simulink model "ELEC448_lab2_dif_kin"  (R2022a)
settings: Solver=ode4  StartTime=0.0  StopTime=inf  FixedStep=0.002  RelTol=1e-3  EnableMultiTasking=on
undefined symbols (not defined in the file or in its folder): HIL, qc_get_step_size
libraries: quarc_library x8
settings Model: ExtModeTrigDuration=10000  Creator=17stf1  LastModifiedBy=19jelg
settings SolverCC: AlgebraicLoopSolver=TrustRegion  PositivePriorityOrder=on
settings DataIOCC: ReturnWorkspaceOutputs=off
settings DebuggingCC: UnconnectedInputMsg=warning  UnconnectedOutputMsg=warning  UnconnectedLineMsg=warning  SFMachineParentedDataDiag=warning  ArithmeticOperatorsInVariantConditions=warning
settings SFSimCC: SimUseLocalCustomCode=off  CustomCodeUndefinedFunction=UseInterfaceOnly
settings RTWCC: Description=QUARC Win64 Target Using Toolchain  SystemTargetFile=quarc_win64.tlc  TemplateMakefile=quarc_default_tmf  RTWUseLocalCustomCode=off  Toolchain=QUARC win64 | nmake (64-bit Windows)  BuildConfiguration=Faster Runs
settings CodeAppCC: StateflowObjectComments=on
settings STFCustomTargetCC: TargetLangStandard=C99 (ISO)  ConcurrentExecutionCompliant=on  UseToolchainInfoCompliant=on  SystemTargetFile=quarc_win64.tlc
settings GRTTargetCC: ParMdlRefBuildCompliant=off  CompOptLevelCompliant=off  CombineOutputUpdateFcns=off  MatFileLogging=off  CPPClassGenCompliant=off  GRTInterface=on  ExtMode=on  ExtModeMexFile=quarc_comm
settings ConfigComp: CovMetricSettings=dswe

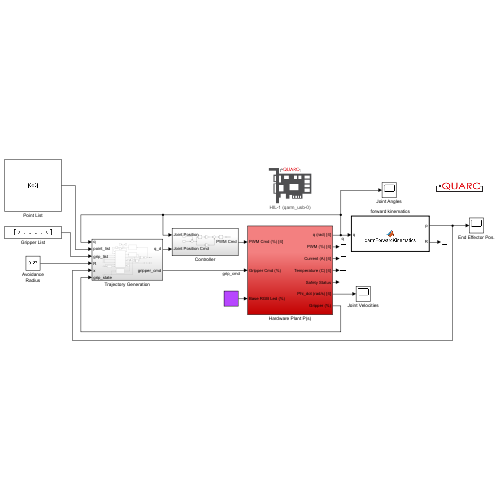
[thumbnail: Simulink's stored preview of the top-level diagram]
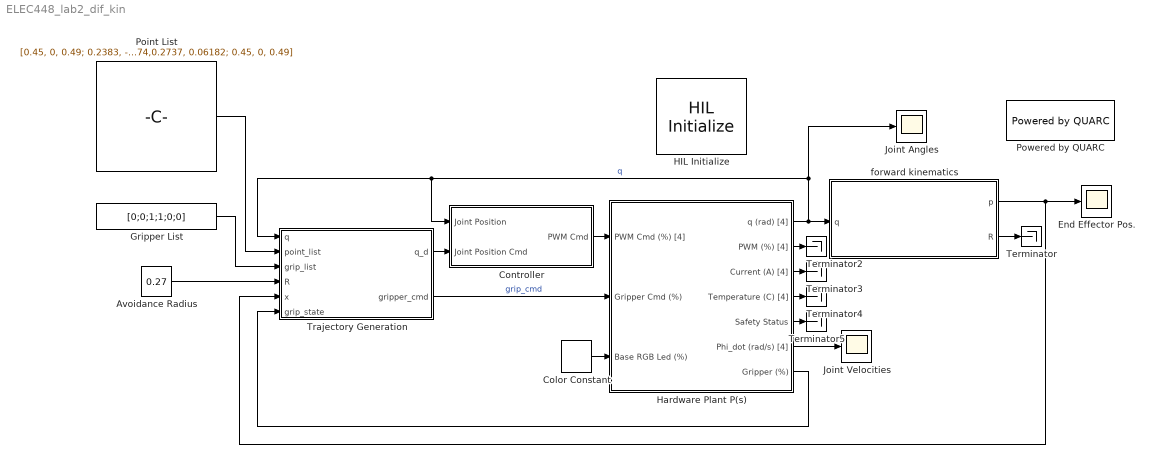
== system ELEC448_lab2_dif_kin ==
  Avoidance Radius : Constant  Value=0.27
  Color Constant : quarc_library/Sources/Signals/Color Constant  color=[0.71765 0.27451 1]
      settings: SourceProductName=QUARC Targets
  Controller : Subsystem
  End Effector Pos. : Scope
  Gripper List : Constant  Value=[0;0;1;1;0;0]
  HIL Initialize : quarc_library/Data Acquisition/Generic/Configuration/HIL Initialize  object_name=HIL-1  board_type=qarm_usb  board_number=0  board_options=j0_mode=1;j1_mode=1;j2_mode=1;j3_mode=1;gripper_mode=0;j0_profile_config=0;j0_profile_velocity=1.5708;j0_profile_acceleration=1.0472;j1_profile_config=0;j1_profile_velocity=1.5708;j1_profile_acceleration=1.0472;j2_profile_config=0;j2_profile_velocity=1.5708;j2_profile_acceleration=1.0472;j3_profile_config=0;j3_profile_velocity=1.5708;j3_profile_acceleration=1.0472;  exclusive=off  active=on  hardware_clocks=[0]  clock_modes=[]  initial_clock_frequencies=[]  set_clock_params_at_start=off  set_clock_params_at_switch_in=off  set_clock_frequencies_at_start=off  set_clock_frequencies_at_switch_in=off  analog_input_channels=[0:9]  analog_input_configurations=[]  analog_input_maximums=5  analog_input_minimums=0  set_analog_input_params_at_start=off  set_analog_input_params_at_switch_in=off  analog_output_channels=[]  analog_output_maximums=[]  analog_output_minimums=[]  initial_analog_outputs=[]  final_analog_outputs=[]  watchdog_analog_outputs=[]  set_analog_output_params_at_start=off  set_analog_output_params_at_switch_in=off  set_analog_outputs_at_start=off  set_analog_outputs_at_switch_in=off  set_analog_outputs_at_terminate=off  set_analog_outputs_at_switch_out=off  set_analog_outputs_on_watchdog=off  digital_input_channels=[]  digital_output_channels=[]  digital_output_configuration=[]  initial_digital_outputs=[0]  final_digital_outputs=[0]  watchdog_digital_outputs=[0]  set_digital_output_params_at_start=off  set_digital_output_params_at_switch_in=off  set_digital_outputs_at_start=on  set_digital_outputs_at_switch_in=off  set_digital_outputs_at_terminate=on  set_digital_outputs_at_switch_out=off  set_digital_outputs_on_watchdog=on  encoder_channels=[]  quadrature=[4]  encoder_filter_frequency=[]  initial_encoder_counts=[0]  set_encoder_params_at_start=off  set_encoder_params_at_switch_in=off  set_encoder_counts_at_start=on  set_encoder_counts_at_switch_in=off  pwm_channels=[]  pwm_modes=[0]  pwm_frequency=50  pwm_configuration=[0]  pwm_alignment=[0]  pwm_polarity=[1]  pwm_leading_deadband=[]  pwm_trailing_deadband=[]  initial_pwm_outputs=[0]  final_pwm_outputs=[0]  watchdog_pwm_outputs=[0]  set_pwm_params_at_start=on  set_pwm_params_at_switch_in=off  set_pwm_outputs_at_start=on  set_pwm_outputs_at_switch_in=off  set_pwm_outputs_at_terminate=on  set_pwm_outputs_at_switch_out=off  set_pwm_outputs_on_watchdog=on  other_output_channels=[1000:1004 11000:11008]  initial_other_outputs=[0]  final_other_outputs=[0]  watchdog_other_outputs=[0]  set_other_outputs_at_start=on  set_other_outputs_at_switch_in=off  set_other_outputs_at_terminate=on  set_other_outputs_at_switch_out=off  set_other_outputs_on_watchdog=on
  Hardware Plant P(s) : Subsystem
  Joint Angles : Scope
  Joint Velocities : Scope
  Point List : Constant  Value=[0.45, 0, 0.49; 0.2383, -0.2831, 0.1474; 0.2379, -0.2736, 0.06678; 0.2593, 0.2566, 0.1446; 0.2574,0.2737, 0.06182; 0.45, 0, 0.49]  VectorParams1D=off
  Powered by QUARC : quarc_library/Logos/Powered by QUARC
  Terminator{,2..5} (5 alike) : Terminator
  Trajectory Generation : Subsystem
  forward kinematics : MATLAB Function  TreatAsAtomicUnit=on
  wires:
  Color Constant/1 -> Hardware Plant P(s)/3(Base RGB Led (%))
  Controller/1(PWM Cmd) -> Hardware Plant P(s)/1(PWM Cmd (%) [4])
  forward kinematics/2(R) -> Terminator/1
  Hardware Plant P(s)/1(q (rad) [4]) -> Joint Angles/1, Controller/1(Joint Position), Trajectory Generation/1(q), forward kinematics/1(q)  "q"
  Trajectory Generation/2(gripper_cmd) -> Hardware Plant P(s)/2(Gripper Cmd (%))  "grip_cmd"
  Hardware Plant P(s)/2(PWM (%) [4]) -> Terminator2/1
  Hardware Plant P(s)/3(Current (A) [4]) -> Terminator3/1
  Hardware Plant P(s)/4(Temperature (C) [4]) -> Terminator4/1
  Hardware Plant P(s)/5(Safety Status) -> Terminator5/1
  Avoidance Radius/1 -> Trajectory Generation/4(R)
  Point List/1 -> Trajectory Generation/2(point_list)
  Gripper List/1 -> Trajectory Generation/3(grip_list)
  Trajectory Generation/1(q_d) -> Controller/2(Joint Position Cmd)
  forward kinematics/1(p) -> Trajectory Generation/5(x), End Effector Pos./1
  Hardware Plant P(s)/7(Gripper (%)) -> Trajectory Generation/6(grip_state)
  Hardware Plant P(s)/6(Phi_dot (rad/s) [4]) -> Joint Velocities/1

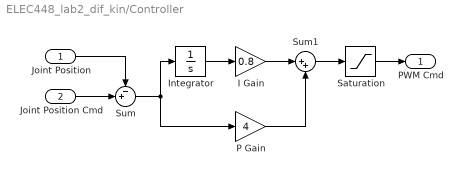
== system ELEC448_lab2_dif_kin/Controller ==
  Joint Position : Inport
  Joint Position Cmd : Inport  Port=2
  I Gain : Gain  Gain=0.8
  Integrator : Integrator  LimitOutput=on  UpperSaturationLimit=0.25  LowerSaturationLimit=-0.25
  P Gain : Gain  Gain=4
  Saturation : Saturate
  Sum : Sum  Inputs=-+|
  Sum1 : Sum  Inputs=|++
  PWM Cmd : Outport
  wires:
  Saturation/1 -> PWM Cmd/1
  Joint Position/1 -> Sum/1
  Joint Position Cmd/1 -> Sum/2
  Integrator/1 -> I Gain/1
  Sum/1 -> P Gain/1, Integrator/1
  Sum1/1 -> Saturation/1
  P Gain/1 -> Sum1/2
  I Gain/1 -> Sum1/1

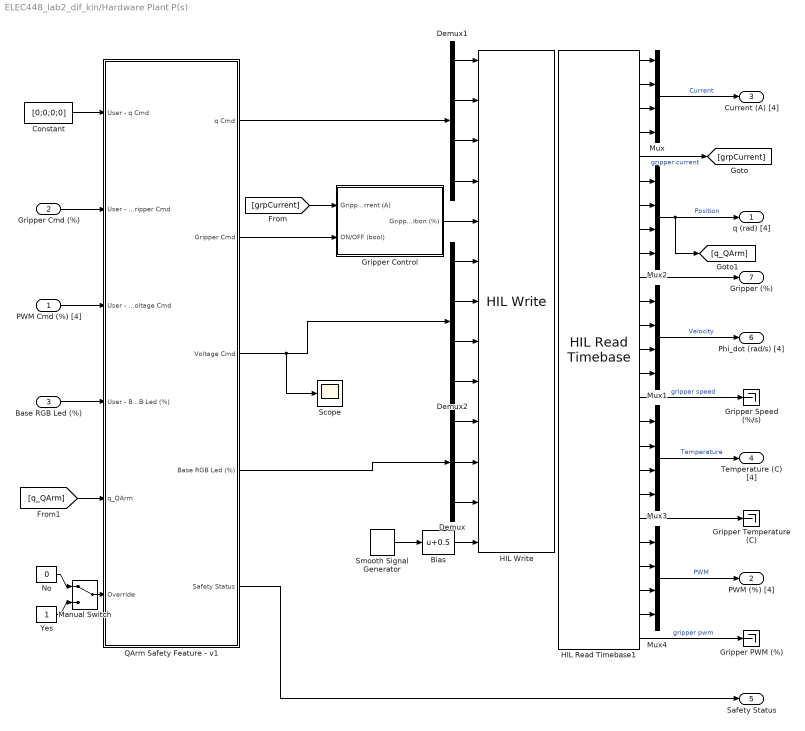
== system ELEC448_lab2_dif_kin/Hardware Plant P(s) ==
  PWM Cmd (%) [4] : Inport
  Gripper Cmd (%) : Inport  Port=2
  Base RGB Led (%) : Inport  Port=3
  Bias : Bias  Bias=0.5  SaturateOnIntegerOverflow=off
  Constant : Constant  Value=[0;0;0;0]
  Demux : Demux  Outputs=3
  Demux1 : Demux
  Demux2 : Demux
  Gripper Control : Subsystem
  Gripper PWM (%) : Terminator
  Gripper Speed (%/s) : Terminator
  Gripper Temperature (C) : Terminator
  HIL Read Timebase1 : quarc_library/Data Acquisition/Generic/Timebases/HIL Read Timebase  object_name=HIL-1  clock=0  analog_channels=[5:9]  encoder_channels=[]  digital_channels=[]  other_channels=[1000:1004 3000:3004 10000:10004 11000:11004]  active=on  vector_output=off  data_type_mode=Inherit via back propagation  encoder_data_type=double  digital_data_type=boolean  overflow_mode=Error on overflow  samples_in_buffer=max(ceil(1/qc_get_step_size), 1)
  HIL Write : quarc_library/Data Acquisition/Generic/Immediate I//O/HIL Write  object_name=HIL-1  analog_channels=[]  pwm_channels=[]  digital_channels=[]  other_channels=[1000:1004 11000:11003 11005:11008]  sample_time=-1  active=on  vector_input=off
  Manual Switch : ManualSwitch
  Mux{,1..4} (5 alike) : Mux
  No : Constant  Value=0
  QArm Safety Feature - v1 : Subsystem
  Scope : Scope
  Smooth Signal Generator : quarc_library/Sources/Signals/Smooth Signal Generator  signal_type=Sine  source=Internal (dialog parameters)  amplitude=0.5  frequency=0.5  initial_phase=0  sample_time=qc_get_step_size  output_cos=off
      settings: SourceProductName=QUARC Targets
  Yes : Constant
  q (rad) [4] : Outport  VectorParamsAs1DForOutWhenUnconnected=off
  PWM (%) [4] : Outport  Port=2  VectorParamsAs1DForOutWhenUnconnected=off
  Current (A) [4] : Outport  Port=3  VectorParamsAs1DForOutWhenUnconnected=off
  Temperature (C) [4] : Outport  Port=4  VectorParamsAs1DForOutWhenUnconnected=off
  Safety Status : Outport  Port=5  VectorParamsAs1DForOutWhenUnconnected=off
  Phi_dot (rad/s) [4] : Outport  Port=6  VectorParamsAs1DForOutWhenUnconnected=off
  Gripper (%) : Outport  Port=7  VectorParamsAs1DForOutWhenUnconnected=off
  wires:
  QArm Safety Feature - v1/2(Gripper Cmd) -> Gripper Control/2(ON/OFF (bool))
  HIL Read Timebase1/10 -> Gripper (%)/1
  Mux4/1 -> PWM (%) [4]/1  "PWM"
  HIL Read Timebase1/25 -> Gripper PWM (%)/1  "gripper pwm"
  HIL Read Timebase1/24 -> Mux4/4
  HIL Read Timebase1/23 -> Mux4/3
  HIL Read Timebase1/22 -> Mux4/2
  HIL Read Timebase1/21 -> Mux4/1
  Demux2/4 -> HIL Write/9
  Demux2/3 -> HIL Write/8
  Demux2/2 -> HIL Write/7
  Demux2/1 -> HIL Write/6
  PWM Cmd (%) [4]/1 -> QArm Safety Feature - v1/3(User - Voltage Cmd)
  Constant/1 -> QArm Safety Feature - v1/1(User - q Cmd)
  Demux1/4 -> HIL Write/4
  Demux1/3 -> HIL Write/3
  Demux1/2 -> HIL Write/2
  Demux1/1 -> HIL Write/1
  Mux3/1 -> Temperature (C) [4]/1  "Temperature"
  Mux1/1 -> Phi_dot (rad/s) [4]/1  "Velocity"
  Mux/1 -> Current (A) [4]/1  "Current"
  HIL Read Timebase1/20 -> Gripper Temperature (C)/1
  HIL Read Timebase1/1 -> Mux/1
  HIL Read Timebase1/2 -> Mux/2
  HIL Read Timebase1/13 -> Mux1/3
  Demux/2 -> HIL Write/11
  HIL Read Timebase1/19 -> Mux3/4
  Demux/1 -> HIL Write/10
  HIL Read Timebase1/11 -> Mux1/1
  HIL Read Timebase1/16 -> Mux3/1
  HIL Read Timebase1/17 -> Mux3/2
  HIL Read Timebase1/3 -> Mux/3
  Demux/3 -> HIL Write/12
  HIL Read Timebase1/15 -> Gripper Speed (%/s)/1  "gripper speed"
  HIL Read Timebase1/5 -> [grpCurrent]  "gripper current"
  HIL Read Timebase1/7 -> Mux2/2
  HIL Read Timebase1/4 -> Mux/4
  HIL Read Timebase1/12 -> Mux1/2
  HIL Read Timebase1/8 -> Mux2/3
  HIL Read Timebase1/18 -> Mux3/3
  HIL Read Timebase1/6 -> Mux2/1
  HIL Read Timebase1/9 -> Mux2/4
  HIL Read Timebase1/14 -> Mux1/4
  Smooth Signal Generator/1 -> Bias/1
  Bias/1 -> HIL Write/13
  Gripper Control/1(Gripper Position (%)) -> HIL Write/5
  [grpCurrent] -> Gripper Control/1(Gripper Current (A))
  [q_QArm] -> QArm Safety Feature - v1/5(q_QArm)
  Yes/1 -> Manual Switch/2
  Manual Switch/1 -> QArm Safety Feature - v1/6(Override)
  No/1 -> Manual Switch/1
  QArm Safety Feature - v1/5(Safety Status) -> Safety Status/1
  QArm Safety Feature - v1/1(q Cmd) -> Demux1/1
  Mux2/1 -> [q_QArm], q (rad) [4]/1  "Position"
  QArm Safety Feature - v1/4(Base RGB Led (%)) -> Demux/1
  Base RGB Led (%)/1 -> QArm Safety Feature - v1/4(User - Base RGB Led (%))
  Gripper Cmd (%)/1 -> QArm Safety Feature - v1/2(User - Gripper Cmd)
  QArm Safety Feature - v1/3(Voltage Cmd) -> Demux2/1, Scope/1

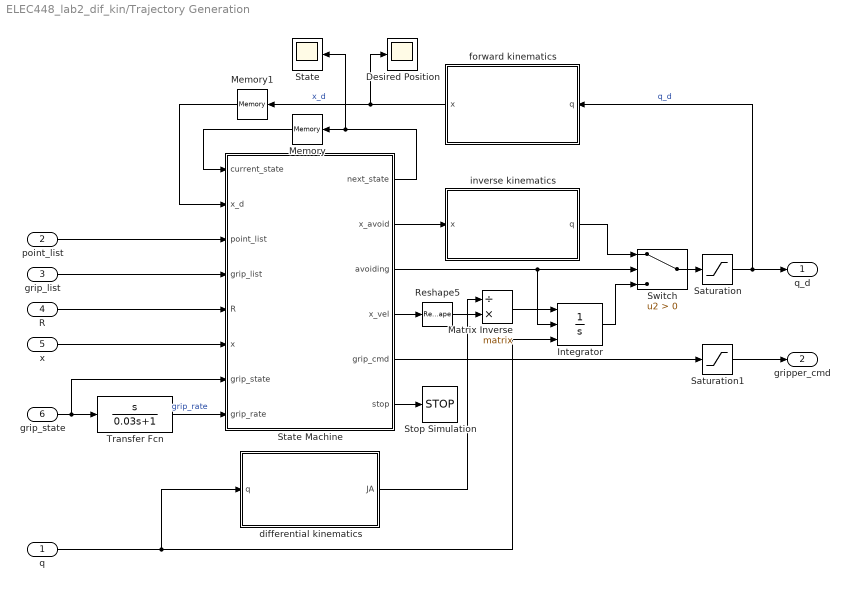
== system ELEC448_lab2_dif_kin/Trajectory Generation ==
  q : Inport
  point_list : Inport  Port=2
  grip_list : Inport  Port=3
  R : Inport  Port=4
  x : Inport  Port=5
  grip_state : Inport  Port=6
  Desired Position : Scope
  Integrator : Integrator  ExternalReset=level  InitialConditionSource=external  UpperSaturationLimit=[170 85 85 180]*pi/180  LowerSaturationLimit=[-170 -85 -95 -180]*pi/180
  Matrix Inverse : Product  Inputs=/*  Multiplication=Matrix(*)
  Memory : Memory  InitialCondition=1
  Memory1 : Memory  InitialCondition=1
  Reshape5 : Reshape  OutputDimensionality=Column vector (2-D)
  Saturation : Saturate  UpperLimit=[170; 85; 75; 167.5]*pi/180  LowerLimit=-[170; 85; 95; 167.5]*pi/180
  Saturation1 : Saturate  UpperLimit=1  LowerLimit=0
  State : Scope
  State Machine : MATLAB Function  TreatAsAtomicUnit=on  SystemSampleTime=0.002
  Stop Simulation : Stop
  Switch : Switch  Criteria=u2 > Threshold  SaturateOnIntegerOverflow=off  InputSameDT=off
  Transfer Fcn : TransferFcn  Numerator=[1 0]  Denominator=[0.03 1]
  differential kinematics : MATLAB Function  TreatAsAtomicUnit=on
  forward kinematics : MATLAB Function  TreatAsAtomicUnit=on
  inverse kinematics : MATLAB Function  TreatAsAtomicUnit=on
  q_d : Outport
  gripper_cmd : Outport  Port=2
  wires:
  forward kinematics/1(x) -> Memory1/1, Desired Position/1  "x_d"
  point_list/1 -> State Machine/3(point_list)
  Memory/1 -> State Machine/1(current_state)
  q/1 -> Integrator/3, differential kinematics/1(q)
  State Machine/4(x_vel) -> Reshape5/1
  R/1 -> State Machine/5(R)
  differential kinematics/1(JA) -> Matrix Inverse/1
  Matrix Inverse/1 -> Integrator/1
  Integrator/1 -> Switch/3
  Saturation/1 -> q_d/1, forward kinematics/1(q)  "q_d"
  State Machine/5(grip_cmd) -> Saturation1/1
  x/1 -> State Machine/6(x)
  Reshape5/1 -> Matrix Inverse/2
  Saturation1/1 -> gripper_cmd/1
  grip_state/1 -> State Machine/7(grip_state), Transfer Fcn/1
  Switch/1 -> Saturation/1
  State Machine/3(avoiding) -> Switch/2, Integrator/2
  State Machine/2(x_avoid) -> inverse kinematics/1(x)
  inverse kinematics/1(q) -> Switch/1
  Memory1/1 -> State Machine/2(x_d)
  State Machine/1(next_state) -> State/1, Memory/1
  grip_list/1 -> State Machine/4(grip_list)
  State Machine/6(stop) -> Stop Simulation/1
  Transfer Fcn/1 -> State Machine/8(grip_rate)  "grip_rate"

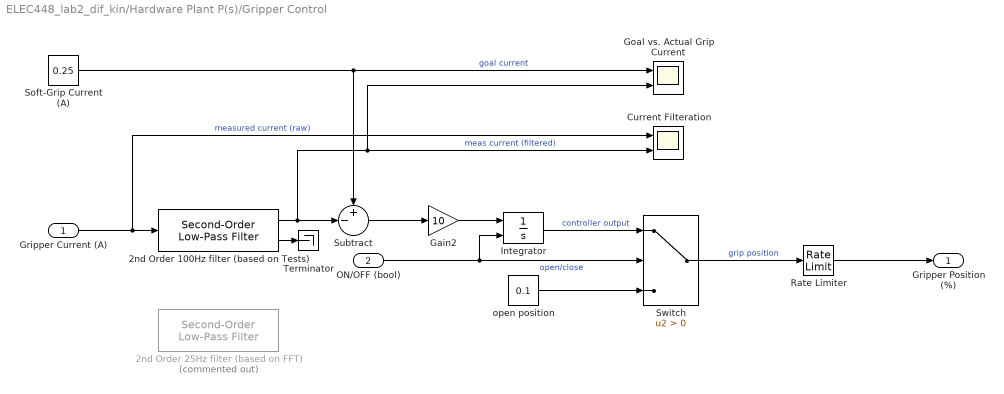
== system ELEC448_lab2_dif_kin/Hardware Plant P(s)/Gripper Control ==
  Gripper Current (A) : Inport
  ON/OFF (bool) : Inport  Port=2
  2nd Order 100Hz filter (based on Tests) : quarc_library/Continuous/Second-Order Low-Pass Filter  params_source=Internal (dialog parameters)  input_width=100*2*pi  input_zeta=1  input_init=0
  2nd Order 25Hz filter (based on FFT) : quarc_library/Continuous/Second-Order Low-Pass Filter  Commented=on  params_source=Internal (dialog parameters)  input_width=25*2*pi  input_zeta=1  input_init=0
  Current Filteration : Scope  NumInputPorts=2
  Gain2 : Gain  Gain=10
  Goal vs. Actual Grip Current : Scope  NumInputPorts=2
  Integrator : Integrator  ExternalReset=either  InitialCondition=0.1  LimitOutput=on  UpperSaturationLimit=0.9  LowerSaturationLimit=0.1
  Rate Limiter : RateLimiter  SampleTimeMode=inherited
  Soft-Grip Current (A) : Constant  Value=0.25
  Subtract : Sum  Inputs=+-|
  Switch : Switch  Criteria=u2 > Threshold  SaturateOnIntegerOverflow=off  InputSameDT=off
  Terminator : Terminator
  open position : Constant  Value=0.1
  Gripper Position (%) : Outport  VectorParamsAs1DForOutWhenUnconnected=off
  wires:
  Gripper Current (A)/1 -> 2nd Order 100Hz filter (based on Tests)/1, Current Filteration/1  "measured current (raw)"
  ON/OFF (bool)/1 -> Switch/2, Integrator/2  "open/close"
  open position/1 -> Switch/3
  Switch/1 -> Rate Limiter/1  "grip position"
  Soft-Grip Current (A)/1 -> Subtract/1, Goal vs. Actual Grip Current/1  "goal current"
  2nd Order 100Hz filter (based on Tests)/1 -> Subtract/2, Current Filteration/2, Goal vs. Actual Grip Current/2  "meas current (filtered)"
  Subtract/1 -> Gain2/1
  Integrator/1 -> Switch/1  "controller output"
  Gain2/1 -> Integrator/1
  2nd Order 100Hz filter (based on Tests)/2 -> Terminator/1
  Rate Limiter/1 -> Gripper Position (%)/1

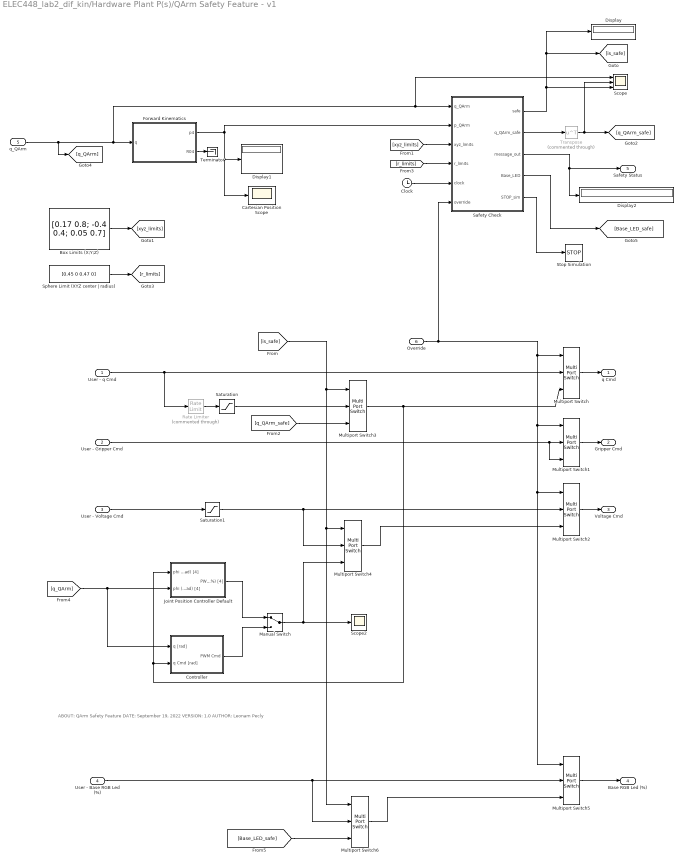
== system ELEC448_lab2_dif_kin/Hardware Plant P(s)/QArm Safety Feature - v1 ==
  note: ABOUT: QArm Safety Feature
      |
      | DATE: September 19, 2022
      |
      | VERSION: 1.0
      |
      | AUTHOR: Leonam Pecly
  User - q Cmd : Inport
  User - Gripper Cmd : Inport  Port=2
  User - Voltage Cmd : Inport  Port=3
  User - Base RGB Led (%) : Inport  Port=4
  q_QArm : Inport  Port=5
  Override : Inport  Port=6
  Box Limits (X;Y;Z) : Constant  Value=[0.17 0.8; -0.4 0.4; 0.05 0.7]
  Cartesian Position Scope : Scope
  Clock : Clock
  Controller : Subsystem
  Display : Display
  Display1 : Display
  Display2 : Display
  Forward Kinematics : MATLAB Function  TreatAsAtomicUnit=on
  Joint Position Controller Default : Subsystem
  Manual Switch : ManualSwitch
  Multiport Switch{,1..6} (7 alike) : MultiPortSwitch  Inputs=2  SaturateOnIntegerOverflow=off  InputSameDT=off
  Rate Limiter : RateLimiter  Commented=through  RisingSlewLimit=pi/2*[1 1 1 2]  FallingSlewLimit=-pi/2*[1 1 1 2]  SampleTimeMode=inherited
  Safety Check : MATLAB Function  TreatAsAtomicUnit=on  SystemSampleTime=qc_get_step_size
  Saturation : Saturate  UpperLimit=pi*[170 85 75 167.5]/180  LowerLimit=pi*[-170 -85 -95 -167.5]/180
  Saturation1 : Saturate  UpperLimit=[1 1 1 1]  LowerLimit=-1*[1 1 1 1]
  Scope : Scope  NumInputPorts=3
  Scope2 : Scope
  Sphere Limit (XYZ center | radius) : Constant  Value=[0.45 0 0.47 0]
  Stop Simulation : Stop
  Terminator : Terminator
  Transpose : Math  Commented=through  Operator=transpose
  q Cmd : Outport
  Gripper Cmd : Outport  Port=2
  Voltage Cmd : Outport  Port=3
  Base RGB Led (%) : Outport  Port=4
  Safety Status : Outport  Port=5
  wires:
  Multiport Switch/1 -> q Cmd/1
  q_QArm/1 -> Scope/1, Safety Check/1(q_QArm), Forward Kinematics/1(q), [q_QArm]
  User - Gripper Cmd/1 -> Multiport Switch1/3, Multiport Switch1/2
  Multiport Switch1/1 -> Gripper Cmd/1
  Multiport Switch2/1 -> Voltage Cmd/1
  User - Voltage Cmd/1 -> Saturation1/1
  Forward Kinematics/1(p4) -> Cartesian Position Scope/1, Display1/1, Safety Check/2(p_QArm)
  [xyz_limits] -> Safety Check/3(xyz_limits)
  Safety Check/1(safe) -> Scope/3, [is_safe], Display/1
  Clock/1 -> Safety Check/5(clock)
  [is_safe] -> Multiport Switch4/1, Multiport Switch6/1, Multiport Switch3/1
  Override/1 -> Safety Check/6(override), Multiport Switch5/1, Multiport Switch2/1, Multiport Switch1/1, Multiport Switch/1
  Box Limits (X;Y;Z)/1 -> [xyz_limits]
  Safety Check/3(message_out) -> Display2/1, Safety Status/1
  [q_QArm] -> Joint Position Controller Default/2(phi (rad) [4]), Controller/1(q [rad])
  User - q Cmd/1 -> Rate Limiter/1, Multiport Switch/2
  Multiport Switch4/1 -> Multiport Switch2/3
  Saturation1/1 -> Multiport Switch2/2, Multiport Switch4/2
  Safety Check/2(q_QArm_safe) -> Transpose/1
  [q_QArm_safe] -> Multiport Switch3/3
  Transpose/1 -> Scope/2, [q_QArm_safe]
  Sphere Limit (XYZ center | radius)/1 -> [r_limits]
  [r_limits] -> Safety Check/4(r_limits)
  Joint Position Controller Default/1(PWM (%) [4]) -> Manual Switch/1
  Controller/1(PWM Cmd) -> Manual Switch/2
  Manual Switch/1 -> Scope2/1, Multiport Switch4/3
  Multiport Switch3/1 -> Multiport Switch/3, Joint Position Controller Default/1(phi cmd (rad) [4]), Controller/2(q Cmd [rad])
  Rate Limiter/1 -> Saturation/1
  Saturation/1 -> Multiport Switch3/2
  Multiport Switch5/1 -> Base RGB Led (%)/1
  User - Base RGB Led (%)/1 -> Multiport Switch5/2, Multiport Switch6/2
  Safety Check/4(Base_LED) -> [Base_LED_safe]
  [Base_LED_safe] -> Multiport Switch6/3
  Multiport Switch6/1 -> Multiport Switch5/3
  Safety Check/5(STOP_sim) -> Stop Simulation/1
  Forward Kinematics/2(R04) -> Terminator/1

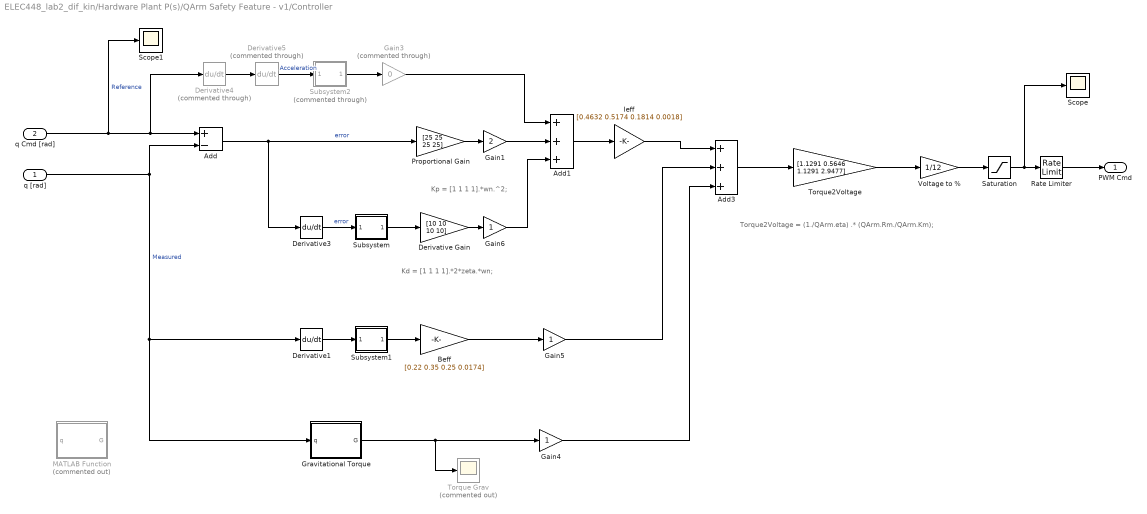
== system ELEC448_lab2_dif_kin/Hardware Plant P(s)/QArm Safety Feature - v1/Controller ==
  note: Kd = [1 1 1 1].*2*zeta.*wn;
  note: Kp = [1 1 1 1].*wn.^2;
  note: Torque2Voltage = (1./QArm.eta) .* (QArm.Rm./QArm.Km);
  q [rad] : Inport
  q Cmd [rad] : Inport  Port=2
  Add : Sum  Inputs=+-
  Add1 : Sum  Inputs=+++
  Add3 : Sum  Inputs=+++
  Beff : Gain  Gain=[0.22 0.35 0.25 0.0174]
  Derivative Gain : Gain  Gain="[10    10    10    10]"
  Derivative1 : Derivative
  Derivative3 : Derivative
  Derivative4 : Derivative  Commented=through
  Derivative5 : Derivative  Commented=through
  Gain1 : Gain  Gain=2
  Gain3 : Gain  Commented=through  Gain=0
  Gain4 : Gain
  Gain5 : Gain
  Gain6 : Gain
  Gravitational Torque : MATLAB Function  TreatAsAtomicUnit=on
  Ieff : Gain  Gain=[0.4632 0.5174 0.1814 0.0018]
  MATLAB Function : MATLAB Function  Commented=on  TreatAsAtomicUnit=on
  Proportional Gain : Gain  Gain="[25    25    25    25]"
  Rate Limiter : RateLimiter  RisingSlewLimit=5*[1 1 1 1]  FallingSlewLimit=-5*[1 1 1 1]  SampleTimeMode=inherited
  Saturation : Saturate  UpperLimit=1  LowerLimit=-1
  Scope : Scope
  Scope1 : Scope
  Subsystem : Subsystem
  Subsystem1 : Subsystem
  Subsystem2 : Subsystem  Commented=through
  Torque Grav : Scope  Commented=on
  Torque2Voltage : Gain  Gain="[1.1291    0.5646    1.1291    2.9477]"
  Voltage to % : Gain  Gain=1/12
  PWM Cmd : Outport
  wires:
  Add/1 -> Proportional Gain/1, Derivative3/1  "error"
  q [rad]/1 -> Add/2, Gravitational Torque/1(q), Derivative1/1  "Measured"
  q Cmd [rad]/1 -> Scope1/1, Add/1, Derivative4/1  "Reference"
  Add3/1 -> Torque2Voltage/1
  Add1/1 -> Ieff/1
  Proportional Gain/1 -> Gain1/1
  Voltage to %/1 -> Saturation/1
  Derivative1/1 -> Subsystem1/1(In1)
  Derivative Gain/1 -> Gain6/1
  Ieff/1 -> Add3/1
  Saturation/1 -> Scope/1, Rate Limiter/1
  Torque2Voltage/1 -> Voltage to %/1
  Derivative4/1 -> Derivative5/1
  Beff/1 -> Gain5/1
  Derivative5/1 -> Subsystem2/1(In1)  "Acceleration"
  Gravitational Torque/1(G) -> Torque Grav/1, Gain4/1
  Gain3/1 -> Add1/1
  Gain4/1 -> Add3/3
  Gain5/1 -> Add3/2
  Gain6/1 -> Add1/3
  Derivative3/1 -> Subsystem/1(In1)  "error"
  Subsystem/1(Out1) -> Derivative Gain/1
  Subsystem1/1(Out1) -> Beff/1
  Subsystem2/1(Out1) -> Gain3/1
  Rate Limiter/1 -> PWM Cmd/1
  Gain1/1 -> Add1/2

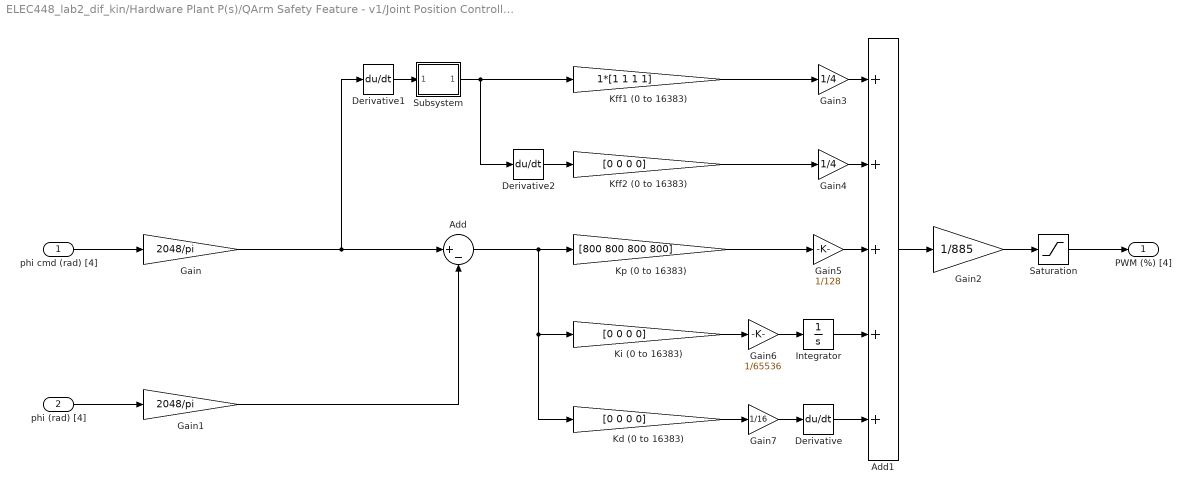
== system ELEC448_lab2_dif_kin/Hardware Plant P(s)/QArm Safety Feature - v1/Joint Position Controller Default ==
  phi cmd (rad) [4] : Inport
  phi (rad) [4] : Inport  Port=2
  Add : Sum  Inputs=|+-
  Add1 : Sum  Inputs=+++++
  Derivative : Derivative
  Derivative1 : Derivative
  Derivative2 : Derivative
  Gain : Gain  Gain=2048/pi
  Gain1 : Gain  Gain=2048/pi
  Gain2 : Gain  Gain=1/885
  Gain3 : Gain  Gain=1/4
  Gain4 : Gain  Gain=1/4
  Gain5 : Gain  Gain=1/128
  Gain6 : Gain  Gain=1/65536
  Gain7 : Gain  Gain=1/16
  Integrator : Integrator
  Kd (0 to 16383) : Gain  Gain=[0 0 0 0]
  Kff1 (0 to 16383) : Gain  Gain=1*[1 1 1 1]
  Kff2 (0 to 16383) : Gain  Gain=[0 0 0 0]
  Ki (0 to 16383) : Gain  Gain=[0 0 0 0]
  Kp (0 to 16383) : Gain  Gain=[800 800 800 800]
  Saturation : Saturate  UpperLimit=[1 1 1 1]  LowerLimit=-1*[1 1 1 1]
  Subsystem : Subsystem
  PWM (%) [4] : Outport  VectorParamsAs1DForOutWhenUnconnected=off
  wires:
  phi cmd (rad) [4]/1 -> Gain/1
  phi (rad) [4]/1 -> Gain1/1
  Gain2/1 -> Saturation/1
  Ki (0 to 16383)/1 -> Gain6/1
  Kd (0 to 16383)/1 -> Gain7/1
  Add/1 -> Kd (0 to 16383)/1, Ki (0 to 16383)/1, Kp (0 to 16383)/1
  Integrator/1 -> Add1/4
  Derivative/1 -> Add1/5
  Add1/1 -> Gain2/1
  Kff2 (0 to 16383)/1 -> Gain4/1
  Derivative1/1 -> Subsystem/1(In1)
  Derivative2/1 -> Kff2 (0 to 16383)/1
  Kff1 (0 to 16383)/1 -> Gain3/1
  Kp (0 to 16383)/1 -> Gain5/1
  Saturation/1 -> PWM (%) [4]/1
  Gain3/1 -> Add1/1
  Gain4/1 -> Add1/2
  Gain5/1 -> Add1/3
  Gain6/1 -> Integrator/1
  Gain7/1 -> Derivative/1
  Gain1/1 -> Add/2
  Gain/1 -> Add/1, Derivative1/1
  Subsystem/1(Out1) -> Derivative2/1, Kff1 (0 to 16383)/1

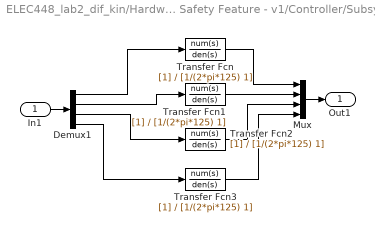
== system ELEC448_lab2_dif_kin/Hardware Plant P(s)/QArm Safety Feature - v1/Controller/Subsystem ==
  In1 : Inport
  Demux1 : Demux
  Mux : Mux
  Transfer Fcn{,1..3} (4 alike) : TransferFcn  Denominator=[1/(2*pi*125) 1]
  Out1 : Outport
  wires:
  Transfer Fcn1/1 -> Mux/2
  Demux1/1 -> Transfer Fcn/1
  Demux1/2 -> Transfer Fcn1/1
  Demux1/3 -> Transfer Fcn2/1
  Transfer Fcn/1 -> Mux/1
  Transfer Fcn3/1 -> Mux/4
  Transfer Fcn2/1 -> Mux/3
  Demux1/4 -> Transfer Fcn3/1
  Mux/1 -> Out1/1
  In1/1 -> Demux1/1

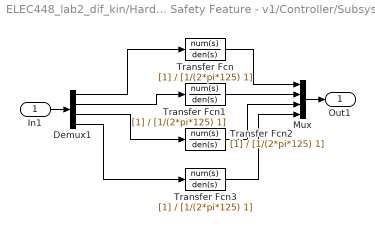
== system ELEC448_lab2_dif_kin/Hardware Plant P(s)/QArm Safety Feature - v1/Controller/Subsystem1 ==
  In1 : Inport
  Demux1 : Demux
  Mux : Mux
  Transfer Fcn{,1..3} (4 alike) : TransferFcn  Denominator=[1/(2*pi*125) 1]
  Out1 : Outport
  wires:
  Transfer Fcn1/1 -> Mux/2
  Demux1/1 -> Transfer Fcn/1
  Demux1/2 -> Transfer Fcn1/1
  Demux1/3 -> Transfer Fcn2/1
  Transfer Fcn/1 -> Mux/1
  Transfer Fcn3/1 -> Mux/4
  Transfer Fcn2/1 -> Mux/3
  Demux1/4 -> Transfer Fcn3/1
  Mux/1 -> Out1/1
  In1/1 -> Demux1/1

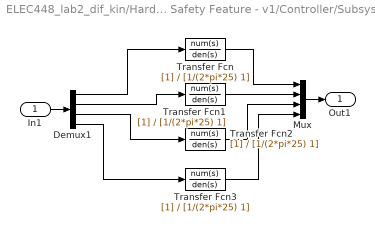
== system ELEC448_lab2_dif_kin/Hardware Plant P(s)/QArm Safety Feature - v1/Controller/Subsystem2 ==
  In1 : Inport
  Demux1 : Demux
  Mux : Mux
  Transfer Fcn{,1..3} (4 alike) : TransferFcn  Denominator=[1/(2*pi*25) 1]
  Out1 : Outport
  wires:
  Transfer Fcn1/1 -> Mux/2
  Demux1/1 -> Transfer Fcn/1
  Demux1/2 -> Transfer Fcn1/1
  Demux1/3 -> Transfer Fcn2/1
  Transfer Fcn/1 -> Mux/1
  Transfer Fcn3/1 -> Mux/4
  Transfer Fcn2/1 -> Mux/3
  Demux1/4 -> Transfer Fcn3/1
  Mux/1 -> Out1/1
  In1/1 -> Demux1/1

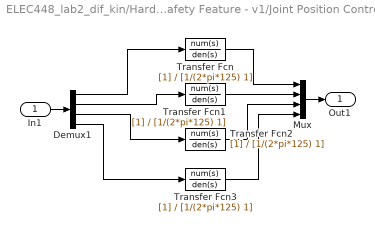
== system ELEC448_lab2_dif_kin/Hardware Plant P(s)/QArm Safety Feature - v1/Joint Position Controller Default/Subsystem ==
  In1 : Inport
  Demux1 : Demux
  Mux : Mux
  Transfer Fcn{,1..3} (4 alike) : TransferFcn  Denominator=[1/(2*pi*125) 1]
  Out1 : Outport
  wires:
  Transfer Fcn1/1 -> Mux/2
  Demux1/1 -> Transfer Fcn/1
  Demux1/2 -> Transfer Fcn1/1
  Demux1/3 -> Transfer Fcn2/1
  Transfer Fcn/1 -> Mux/1
  Transfer Fcn3/1 -> Mux/4
  Transfer Fcn2/1 -> Mux/3
  Demux1/4 -> Transfer Fcn3/1
  Mux/1 -> Out1/1
  In1/1 -> Demux1/1

== matlab function ELEC448_lab2_dif_kin/Trajectory Generation/forward kinematics ==
  data: q input; x output
function x  = qarmForwardKinematics(q)

%% QUANSER_ARM_FPK
% v 4.0 - 4th June 2020
% Modified for ELEC 448 by Shane Forbrigger - March 6 2021

% REFERENCE: 
% Chapter 3. Forward Kinematics
% Robot Dynamics and Control 
% Spong, Vidyasagar
% 1989

% INPUTS:
% q       : Alternate joint angles vector 4 x 1

% OUTPUTS:
% p4      : End-effector frame {4} position vector expressed in base frame {0}
% R04     : rotation matrix from end-effector frame {4} to base frame {0}

%% Manipulator parameters:
L1 = 0.1400;
L2 = 0.3500;
L3 = 0.0500;
L4 = 0.2500;
L5 = 0.1500;

%% Alternate parameters
l1 = L1;
l2 = sqrt(L2^2 + L3^3);
l3 = L4 + L5;
beta = atan(L3/L2);

%% From q space to theta space 
theta = q - [0; pi/2-beta; beta; 0];

%% Position of end-effector Transformation
c = cos(theta);
s = sin(theta);
c23 = cos(theta(2) + theta(3));
s23 = sin(theta(2) + theta(3));
% Calculate the Position vector 
x = [c(1)*(l2*c(2) - l3*s23);
     s(1)*(l2*c(2) - l3*s23);
     l1 - l2*s(2) - l3*c23;
     theta(4)];

end

== matlab function ELEC448_lab2_dif_kin/Trajectory Generation/inverse kinematics ==
  data: q output; x input
function q   = qarmInverseKinematics(x)

%% QUANSER_ARM_IPK
% v 4.0 - 4th June 2020
% Modified by Shane Forbrigger for ELEC 448 - March 7 2021

% REFERENCE: 
% Chapter 4. Inverse Kinematics
% Robot Dynamics and Control 
% Spong, Vidyasagar
% 1989

% INPUTS:
% p   : The end-effector position vector expressed in base frame {0}.

% OUTPUTS:
% phi : The inverse kinematics solution: a [4x1] vector of joint 
%       angles.

%% Manipulator parameters:
L1 = 0.1400;
L2 = 0.3500;
L3 = 0.0500;
L4 = 0.2500;
L5 = 0.1500;

%% Alternate parameters
l1 = L1;
l2 = sqrt(L2^2 + L3^3);
l3 = L4 + L5;
beta = atan(L3/L2);

%% Initialization
theta = zeros(4,1);
q = zeros(4,1);

%% Joint angle 1: 
theta(1) = atan2(x(2),x(1));
%% Position relative to frame 1
p1 = [norm(x(1:2)); l1 - x(3); 0];
gamma = -atan(p1(2)/p1(1));
%% Joint angle 2:
theta(2) = -acos((l2^2 - l3^2 + norm(p1)^2)/(2*l2*norm(p1))) - gamma;
%% Joint angle 3
theta(3) = asin((l2^2 + l3^2 - norm(p1)^2)/(2*l2*l3));
%% Joint angle 4
theta(4) = x(4);
%% Remap theta back to phi
q = theta + [0; pi/2-beta; beta; 0];


end

== matlab function ELEC448_lab2_dif_kin/forward kinematics ==
  data: q input; p output; R output
function [p, R] = qarmForwardKinematics(q)

%% QUANSER_ARM_FPK
% v 4.0 - 4th June 2020
% Modified for ELEC 448 by Shane Forbrigger - March 6 2021

% REFERENCE: 
% Chapter 3. Forward Kinematics
% Robot Dynamics and Control 
% Spong, Vidyasagar
% 1989

% INPUTS:
% q     : Alternate joint angles vector 4 x 1

% OUTPUTS:
% p      : End-effector frame {4} position vector expressed in base frame {0}
% R     : rotation matrix from end-effector frame {4} to base frame {0}

%% Manipulator parameters:
L1 = 0.1400;
L2 = 0.3500;
L3 = 0.0500;
L4 = 0.2500;
L5 = 0.1500;

%% Alternate parameters
l1 = L1;
l2 = sqrt(L2^2 + L3^3);
l3 = L4 + L5;
beta = atan(L3/L2);

%% From q space to theta space 
theta = q - [0; pi/2-beta; beta; 0];

%% Position of end-effector Transformation
c = cos(theta);
s = sin(theta);
c23 = cos(theta(2) + theta(3));
s23 = sin(theta(2) + theta(3));
% Calculate the Position vector 
p = [c(1)*(l2*c(2) - l3*s23);
     s(1)*(l2*c(2) - l3*s23);
     l1 - l2*s(2) - l3*c23];

% Calculate the Rotation matrix
R = [c(1)*c23*c(4) + s(1)*s(4), -c(1)*c23*s(4) + s(1)*c(4), -c(1)*s23;
     s(1)*c23*c(4) - c(1)*s(4), -s(1)*c23*s(4) - c(1)*c(4), -s(1)*s23;
    -s23*c(4), s23*s(4), -c23];

end

== matlab function ELEC448_lab2_dif_kin/Hardware Plant P(s)/QArm Safety Feature - v1/Controller/Gravitational Torque ==
  data: q input; G output
function G = tau_g(q)

g = 9.81;
L2 = 0.3500;
L3 = 0.0500;
L4 = 0.2500;
L5 = 0.1500;
beta = atan(L3/L2);
theta = q(1,1:4) - [0, pi/2-beta, beta, 0];    % Maps Phi to Theta

m2 = 0.4591;
m3 = 0.269;
m4 = 0.257;
lc2 = 0.1071;
lc3 = 0.1561;
lc4 = 0.0998;
l2 = sqrt(L2^2 + L3^2);         % lambda 2
l3 = L4 + L5;                   % lambda 3
%% Gravitational Terms
G1 = 0;
G2 = -g*(m2*(l2 - lc2)*cos(theta(2)) + m3*(l2*cos(theta(2)) - lc3*sin(theta(2)+theta(3))) + m4*(l2*cos(theta(2)) - (l3 - lc4)*sin(theta(2)+theta(3))) );
G3 = g*(m3*lc3*sin(theta(2)+theta(3)) + m4*(l3 - lc4)*sin(theta(2)+theta(3)) );
G4 = 0;

G = [G1, G2, G3, G4];

== matlab function ELEC448_lab2_dif_kin/Hardware Plant P(s)/QArm Safety Feature - v1/Controller/MATLAB Function ==
  data: q input; G output
function G = tau_g(q)

g = 9.81;
L2 = 0.3500;
L3 = 0.0500;
L4 = 0.2500;
L5 = 0.1500;
beta = atan(L3/L2);
theta = q - [0, pi/2-beta, beta, 0];    % Maps Phi to Theta

m2 = 0.4591;
m3 = 0.269;
m4 = 0.257;
lc2 = 0.1071;
lc3 = 0.1561;
lc4 = 0.0998;
l2 = sqrt(L2^2 + L3^2);         % lambda 2
l3 = L4 + L5;                   % lambda 3
mL = 0;

G2 = -g*(m2*(l2 - lc2)*cos(theta(2)) + m3*(l2*cos(theta(2)) - lc3*sin(theta(2)+theta(3))) + m4*(l2*cos(theta(2)) - (l3 - lc4)*sin(theta(2)+theta(3))) + mL*(l2*cos(theta(2)) - l3*sin(theta(2)+theta(3))) );
G3 = g*(m3*lc3*sin(theta(2)+theta(3)) + m4*(l3 - lc4)*sin(theta(2)+theta(3)) + mL*l3*sin(theta(2)+theta(3)) );

G = [0, G2, G3, 0];

== matlab function ELEC448_lab2_dif_kin/Hardware Plant P(s)/QArm Safety Feature - v1/Forward Kinematics ==
  data: q input; p4 output; R04 output
function [p4, R04] = qarmForwardKinematics(q)

%% QUANSER_ARM_FPK
% v 4.0 - 4th June 2020
% Code updated by Leonam Pecly - August 5, 2021

% REFERENCE: 
% Chapter 3. Forward Kinematics
% Robot Dynamics and Control 
% Spong, Vidyasagar
% 1989

% INPUTS:
% phi     : Alternate joint angles vector 4 x 1

% OUTPUTS:
% p4      : End-effector frame {4} position vector expressed in base frame {0}
% R04     : rotation matrix from end-effector frame {4} to base frame {0}

%% Manipulator parameters:
L1 = 0.1400;
L2 = 0.3500;
L3 = 0.0500;
L4 = 0.2500;
L5 = 0.1500;

%% Alternate parameters (Quanser QArm-Lab2 - Table 2 - left)
l1 = L1;
l2 = sqrt(L2^2 + L3^2);
l3 = L4 + L5;
beta = atan(L3/L2);

%% From phi space to theta space (Quanser QArm-Lab2 - Table 2 - right)
theta = q - [0; pi/2-beta; beta; 0];

%% Transformation matrices for all frames:

% % T{i-1}{i} = quanser_arm_DH(  a, alpha,  d,     theta );
%         T01 = quanser_arm_DH(  0,     0,  0,         0 );
%         T12 = quanser_arm_DH(  0,     0,  0,         0 );
%         T23 = quanser_arm_DH(  0,     0,  0,         0 );
%         T34 = quanser_arm_DH(  0,     0,  0,         0 );
% 
%         T02 = ;
%         T03 = ;
%         T04 = ;

%% Position of end-effector Transformation
s23 = sin(theta(2) + theta(3));

% Position vector 
p4 =  [-cos(theta(1))*(l3*s23 - l2*cos(theta(2)));
       -sin(theta(1))*(l3*s23 - l2*cos(theta(2)));
       l1 - l3*cos(theta(2) + theta(3)) - l2*sin(theta(2))];
% Rotation matrix
R04 = zeros(3,3);

end

% % 
% % function T = quanser_arm_DH(a,alpha,d,theta)
% % 
% % %% QUANSER_ARM_DH
% % % v 1.0 - 26th March 2019
% % 
% % % REFERENCE: 
% % % Chapter 3. Forward and Inverse Kinematics
% % % Robot Modeling and Control 
% % % Spong, Hutchinson, Vidyasagar
% % % 2006
% % 
% % % INPUTS:
% % % a       :   translation  : along : x_{i}   : from : z_{i-1} : to : z_{i}
% % % alpha   :      rotation  : about : x_{i}   : from : z_{i-1} : to : z_{i}
% % % d       :   translation  : along : z_{i-1} : from : x_{i-1} : to : x_{i}
% % % theta   :      rotation  : about : z_{i-1} : from : x_{i-1} : to : x_{i}
% % % NOTE: Standard DH Parameters
% % 
% % % OUTPUTS:
% % % T       : transformation                   : from :     {i} : to : {i-1}
% % 
% % %%
% % % Rotation Transformation about z axis by theta
% % T_R_z = [cos(theta) -sin(theta) 0 0;
% %       sin(theta) cos(theta) 0 0;
% %       0 0 1 0;
% %       0 0 0 1];
% %      
% % % Translation Transformation along z axis by d
% % T_T_z = [1 0 0 0; 0 1 0 0; 0 0 1 d; 0 0 0 1];
% % 
% % % Translation Transformation along x axis by a
% % T_T_x = [1 0 0 a; 0 1 0 0; 0 0 1 0; 0 0 0 1];;
% % 
% % % Rotation Transformation about x axis by alpha
% % T_R_x = [1 0 0 0;
% %       0 cos(alpha) -sin(alpha) 0;
% %       0 sin(alpha) cos(alpha) 0;
% %       0 0 0 1];
% % 
% % % For a transformation FROM frame {i} TO frame {i-1}:
% % % rotate about z
% % % then translate along z, 
% % % then translate along x, 
% % % then rotate about x, 
% % 
% % T = Rz*Tz*Tx*Rx;
% % 
% % end

== matlab function ELEC448_lab2_dif_kin/Hardware Plant P(s)/QArm Safety Feature - v1/Safety Check ==
  data: q_QArm input; p_QArm input; safe output; xyz_limits input; r_limits input; clock input; q_QArm_safe output; message_out output; Base_LED output; override input; STOP_sim output
function [safe,q_QArm_safe,message_out,Base_LED,STOP_sim] = fcn(q_QArm,p_QArm,xyz_limits,r_limits,clock,override)
% ABOUT: Safety Check
% DATE: September 19, 2022
% VERSION: 1.0
% Author: Leonam Pecly

q_home_position = [0 0 0 0]';

persistent is_position_safe clock_not_safe q_QArm_not_safe message%is_cmd_safe
if isempty(is_position_safe)
    %is_cmd_safe = 1;
    is_position_safe = 1; % 1 = is safe | 0 = NOT safe
    clock_not_safe = 0;
    q_QArm_not_safe = q_home_position;
    message = "-------- Initialization --------";
    message_add = "         ";
end

%% Safety Check
if (is_position_safe)
    if (override < 0.5) % Do not check if override is ON
        safe = f_check_rules(q_QArm,p_QArm);
        is_position_safe = safe;
        message = "Ok";
    else
        safe = is_position_safe;
        message = "Override";
    end
    
    Base_LED = [0 0 0];
else
    safe = 0;
    Base_LED = [1 0 0] * sin(2*pi*clock); % Red blinking at 1 Hz
    message = "Danger";
end

STOP_sim = 0;
%% Safe Position
if (is_position_safe)
    q_QArm_safe = q_QArm;

else % Return to Home
    if (clock_not_safe == 0) % Run just once
        clock_not_safe = clock;
        q_QArm_not_safe = q_QArm;
    end

    if (clock <= clock_not_safe+1) % Stop and Wait 1 s
        q_QArm_safe = q_QArm_not_safe;
    elseif (clock <= clock_not_safe+3)
        % Exponential decay returning home
        q_QArm_safe = q_QArm_not_safe * exp(2.5*(clock_not_safe+1 - clock)); %
    elseif (clock <= clock_not_safe+8) % Wait 5 s
        q_QArm_safe = q_home_position;
    else
        q_QArm_safe = q_home_position;
        STOP_sim = 1;
    end
end

%% Message

message_out = message;

%% Check Rules
function check = f_check_rules(joint_QArm,EE_QArm)
    
    % QArm joint limits
    if (joint_QArm(1) > 170*pi/180 || joint_QArm(1) < -170*pi/180 ...
        || joint_QArm(2) > 80*pi/180 || joint_QArm(2) < -80*pi/180 ...
        || joint_QArm(3) > 75*pi/180 || joint_QArm(3) < -95*pi/180 ...
        || joint_QArm(4) > 160*pi/180 || joint_QArm(4) < -160*pi/180)
        
        check = 0; % NOT Ok
        return;
    else
        check = 1; % Ok
    end    
    
    %Box limits
    if ((EE_QArm(1) >= xyz_limits(1,1)) && (EE_QArm(1) <= xyz_limits(1,2)) &&...
        (EE_QArm(2) >= xyz_limits(2,1)) && (EE_QArm(2) <= xyz_limits(2,2)) &&...
        (EE_QArm(3) >= xyz_limits(3,1)) && (EE_QArm(3) <= xyz_limits(3,2))...
        )
        check = 1; % Ok
    else
        check = 0; % NOT Ok
        return;
    end

    %Sphere limits
    if (r_limits(4) > 0)
        distance = norm(EE_QArm - r_limits(1:3));
        if (distance < r_limits(4))
            check = 1; % Ok
        else
            check = 0; % NOT Ok

            return;
        end        
    end

end

end

== matlab function ELEC448_lab2_dif_kin/Trajectory Generation/State Machine ==
  data: current_state input; x_d input; next_state output; x_avoid output; avoiding output; point_list input; grip_list input; R input; x input; grip_state input; grip_rate input; x_vel output; grip_cmd output; stop output
function [next_state, x_avoid, avoiding, x_vel,  grip_cmd, stop] = stateMachine(current_state, x_d, point_list, grip_list, R, x, grip_state, grip_rate)

persistent target theta_f
if isempty(target)
    target = 1;
    theta_f = nan;
end
% Desired velocity magnitude for the robot's end-effector motion
v_mag = 0.25; % [m/s]
% We want to be within a centimetre of the target, but our precision 
% is limited by the velocity and sample time
error_tolerance = max(0.01, 1.1*v_mag*0.002);
% It is sufficient for the robot to be within 5 degrees of the exit point
% for the singularity avoidance trajectory
theta_tolerance = deg2rad(5);
% Error between the current robot position and the target
target_error = point_list(target,:)' - x(1:3);
% The singularity avoidance region is a cylinder surrounding Joint 1's axis
insideCircle = norm(x_d(1:2),2) <= R;
% Boolean to stop the simulation after all targets have been reached
stop = 0;

% If this is the first target, the gripper should be open until the robot
% transitions into the opening/closing state. Otherwise, it should maintain
% the previous grip command
if target == 1
    grip_cmd = 0;
else
    grip_cmd = grip_list(target-1);
end

x_avoid = zeros(4,1);

switch current_state
    % Beelining to target position
    case 1
        % Creating a velocity vector that points to the target
        x_vel = [v_mag*target_error/(norm(target_error) + 0.001); 0];
        next_state = current_state;
        avoiding = 0;
        % If the robot reaches near the target
        if norm(target_error) < error_tolerance
            % Stop the robot
            x_vel = 0*x_vel;
            next_state = 3;
        % Setting up avoidance trajectory if in the circle and not leaving
        elseif insideCircle && dot(target_error,x_d(1:3)) < 0
            % Starting point on the avoidance trajectory
            x_i = [x_d(1:2); 0];
            % Error vector in the x-y plane to the target point
            xy_error = [target_error(1:2); 0];
            % Length of the straight-line trajectory passing through the avoidance region
            L = 2*abs(dot(x_i, xy_error))/norm(xy_error);
            % Starting angle of the avoidance trajectory around the 
            % avoidance region
            theta_i = atan2(x_i(2),x_i(1));
            % Magnitude of the angle from the starting point on the
            % cylinder to the end point on the cylinder
            theta_max = 2*asin(0.5*L/R);
            % Calculate the direction to move around the avoidance region
            rot_direction = cross(xy_error,-x_i);
            rot_direction = sign(rot_direction(3));
            % Ensuring the final angle is within -pi to pi
            theta_f = mod(theta_i + rot_direction*theta_max + pi, 2*pi) - pi;
            % Stop the robot
            x_vel = 0*x_vel;
            next_state = 2;
        end
    % Avoiding singularity
    case 2
        avoiding = 1;
        x_vel = [0; 0; 0; 0];
        x_avoid = x_d;
        % The current angle of the avoidance trajectory relative to z-axis
        theta_current = atan2(x_d(2),x_d(1));
        % The error between the current angle and the final angle of the
        % avoidance trajectory
        delta_theta = theta_f - theta_current;
        % If the robot is near the end of the avoidance trajectory
        if abs(delta_theta) < theta_tolerance
            % Move the robot in a straight line to the target
            x_vel = [v_mag*target_error/(norm(target_error) + 0.001); 0];
            next_state = 1;
            avoiding = 0;
        else
            % Move the robot around the edge of the avoidance region for
            % one time step
            theta_next = theta_current + 0.002*sign(delta_theta)*v_mag/R;
            x_avoid(1:2) = R*[cos(theta_next); sin(theta_next)];
            next_state = current_state;
        end
    % Opening/closing gripper
    case 3
        x_vel = [0; 0; 0; 0];
        avoiding = 0;
        grip_cmd = grip_list(target);
        % If the gripper is near the target and changing less than 1%/second
        if (abs(grip_state - grip_cmd) < 0.5) && (abs(grip_rate) < 0.01)
            next_state = 1;
            N_points = size(point_list,1);
            % Change to the next target point
            target = target + 1;
            % Stop the simulation if the last target was reached
            if target > N_points
                stop = 1;
            end
        else
            next_state = current_state;
        end
        
	% Default Case
    otherwise
        % State Transition
        next_state = current_state;    
        % State Action
        x_vel = [0; 0; 0; 0];
        grip_cmd = 0;
        avoiding = 0;
end

== matlab function ELEC448_lab2_dif_kin/Trajectory Generation/differential kinematics ==
  data: q input; JA output
function JA   = qarmDifferentialKinematics(q)

%% QUANSER_ARM_FDK
% v 1.0 - 13th August 2020

% REFERENCE: 
% Chapter 5. Velocity Kinematics
% Robot Dynamics and Control 
% Spong, Vidyasagar
% 1989

% INPUTS:
% q : Joint angles (4x1 vector) output by the robot in RADIANS

% OUTPUTS:
% JA : The analytical Jacobian matrix (4x4 matrix) relating the end
%      effector linear velocity and roll angular velocity to the angular
%      velocity of the joints.

%% Manipulator parameters:
L1 = 0.1400;
L2 = 0.3500;
L3 = 0.0500;
L4 = 0.2500;
L5 = 0.1500;

%% Alternate parameters
% Each lowercase l represents "lambda" from the lab manual
l1 = L1;
l2 = sqrt(L2^2 + L3^2);
l3 = L4 + L5;
beta = atan(L3/L2);

%% From q space to theta space 
theta = q - [0; pi/2-beta; beta; 0];

%% Jacobian term definition:
% Use the following variable definitions to help you write simpler code.
% "c" and "s" are the sine and cosine of theta. Each is a vector where the
% ith element represents cos(theta(i)) or sin(theta(i)). "c23" and "s23"
% are single-element variables that represent the cosine and sine of the
% sum of the angles for joints 2 and 3.
s = sin(theta);
c = cos(theta);
s23 = sin(theta(2) + theta(3));
c23 = cos(theta(2) + theta(3));

JA = eye(4);
JA(1,1) = -s(1)*(l2*c(2)-l3*s23); 
JA(1,2) = c(1)*(-l2*s(2)-l3*c23); 
JA(1,3) = -l3*c(1)*c23; 
JA(2,1) = c(1)*(l2*c(2)-l3*s23); 
JA(2,2) = s(1)*(-l2*s(2)-l3*c23);
JA(2,3) = -l3*s(1)*c23;
JA(3,1) = 0;
JA(3,2) = -l2*c(2)+l3*s23;
JA(3,3) = l3*s23;

end
